simulink model "Simulink_P6"  (R2025b)
settings: Solver=VariableStepAuto  StartTime=0.0  StopTime=0.010  RelTol=1e-3
InitFcn:
  | L = 2e-3;
  | R = 10;
  | C = 10e-6;
  | Vin = 32;

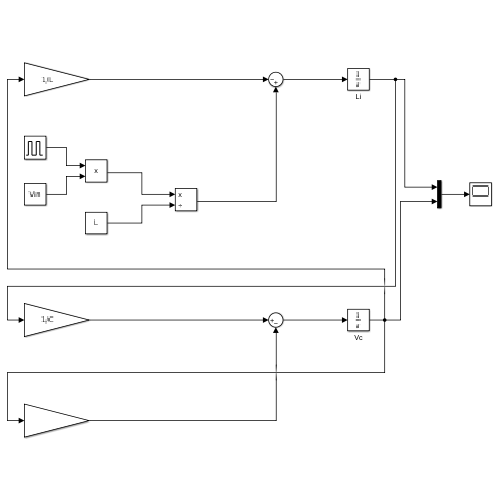
[thumbnail: Simulink's stored preview of the top-level diagram]
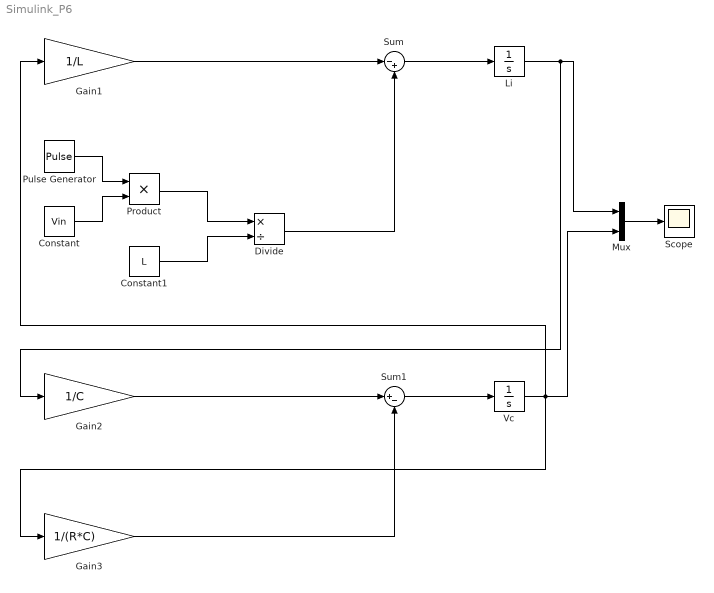
== system Simulink_P6 ==
  Constant : Constant  Value=Vin
  Constant1 : Constant  Value=L
  Divide : Product  Inputs=*/
  Gain1 : Gain  Gain=1/L
  Gain2 : Gain  Gain=1/C
  Gain3 : Gain  Gain=1/(R*C)
  Li : Integrator
  Mux : Mux  Inputs=2
  Product : Product
  Pulse Generator : DiscretePulseGenerator  PulseType=Time based  Period=1/100e3  PulseWidth=40
  Scope : Scope
      settings: ActiveDisplayYMinimum=0.22059018705030198  ActiveDisplayYMaximum=14.787681926463538
  Sum : Sum  Inputs=|-+
  Sum1 : Sum  Inputs=|+-
  Vc : Integrator
  wires:
  Pulse Generator/1 -> Product/1
  Constant/1 -> Product/2
  Product/1 -> Divide/1
  Constant1/1 -> Divide/2
  Gain1/1 -> Sum/1
  Divide/1 -> Sum/2
  Sum/1 -> Li/1
  Gain2/1 -> Sum1/1
  Gain3/1 -> Sum1/2
  Sum1/1 -> Vc/1
  Mux/1 -> Scope/1
  Li/1 -> Gain2/1, Mux/1
  Vc/1 -> Gain3/1, Gain1/1, Mux/2
